simulink model "TP3_LABO_CONTROL_real_marcos"  (R2024b)
settings: Solver=VariableStepAuto  StartTime=0.0  StopTime=20  FixedStep=0.02  RelTol=1e-3
values from neighbouring files (symbols this model uses):
  Ad = eye(size(A)) + Ts * A    [observador_balta.m]    (also in observador_balta_2.m)
  Bd = Ts * B    [observador_balta.m]    (also in observador_balta_2.m)
  Cd = C    [observador_balta.m]    (also in observador_balta_2.m)
  K = K_scaled * T_inv    [real_estados_balta.m]    (also in todoslospuntos.m = -b * p / (1 - exp(-p * Ts)))
  L = P1*C    [estimacion_ecuaciones.m]    (also in observador_balta.m = P1*C1; observador_balta_2.m = P1*C1; real_estados_balta.m = T * L_scaled)
  Ts = 0.01    [Codigos_acomodados_14_5.m]    (also in PlantaEstable.m = median(diff(t_rec)); estimacion_ecuaciones.m; observador_balta.m = 0.02; observador_balta_2.m = 0.02)
undefined symbols (not defined in the file or in its folder): Kint
settings Model: Creator=lococ  LastModifiedBy=lococ

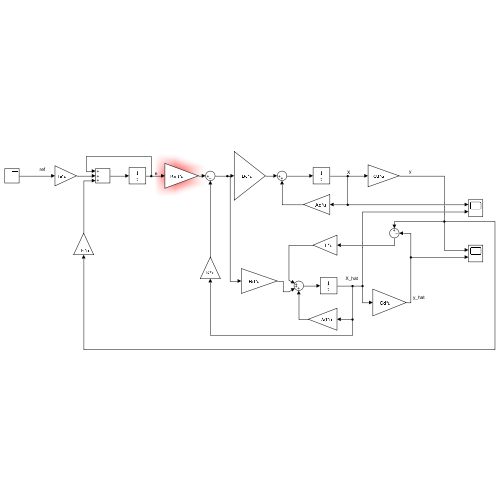
[thumbnail: Simulink's stored preview of the top-level diagram]
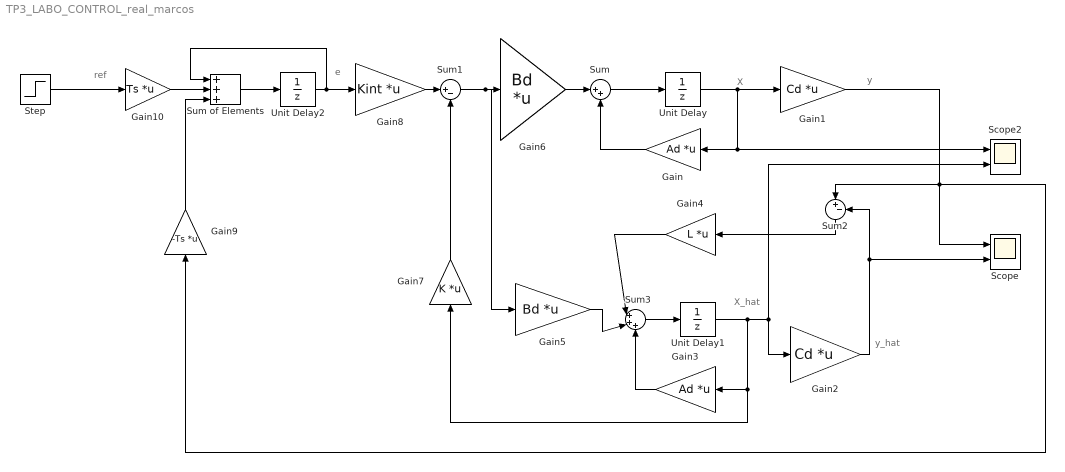
== system TP3_LABO_CONTROL_real_marcos ==
  note: ref
  note: e
  note: X_hat
  note: y_hat
  note: y
  note: X
  Gain : Gain  Gain=Ad  Multiplication=Matrix(K*u)
  Gain1 : Gain  Gain=Cd  Multiplication=Matrix(K*u)
  Gain10 : Gain  Gain=Ts  Multiplication=Matrix(K*u)
  Gain2 : Gain  Gain=Cd  Multiplication=Matrix(K*u)
  Gain3 : Gain  Gain=Ad  Multiplication=Matrix(K*u)
  Gain4 : Gain  Gain=L  Multiplication=Matrix(K*u)
  Gain5 : Gain  Gain=Bd  Multiplication=Matrix(K*u)
  Gain6 : Gain  Gain=Bd  Multiplication=Matrix(K*u)
  Gain7 : Gain  Gain=K  Multiplication=Matrix(K*u)
  Gain8 : Gain  Gain=Kint  Multiplication=Matrix(K*u)
  Gain9 : Gain  Gain=-Ts  Multiplication=Matrix(K*u)
  Scope : Scope  NumInputPorts=2
  Scope2 : Scope  NumInputPorts=2
  Step : Step  Time=[1;1]  Before=[0;0]  After=[30;0]  SampleTime=0  VectorParams1D=off
  Sum : Sum  Inputs=|++
  Sum of Elements : Sum  Inputs=+++
  Sum1 : Sum  Inputs=|+-
  Sum2 : Sum  Inputs=|+-
  Sum3 : Sum  Inputs=|+++
  Unit Delay : UnitDelay  SampleTime=0.02  HasFrameUpgradeWarning=on
  Unit Delay1 : UnitDelay  SampleTime=0.02  HasFrameUpgradeWarning=on
  Unit Delay2 : UnitDelay  SampleTime=0.02  HasFrameUpgradeWarning=on
  wires:
  Sum/1 -> Unit Delay/1
  Gain/1 -> Sum/2
  Unit Delay/1 -> Scope2/1, Gain/1, Gain1/1
  Gain2/1 -> Sum2/2, Scope/2
  Sum2/1 -> Gain4/1
  Gain4/1 -> Sum3/1
  Gain3/1 -> Sum3/3
  Gain5/1 -> Sum3/2
  Gain6/1 -> Sum/1
  Sum1/1 -> Gain5/1, Gain6/1
  Gain7/1 -> Sum1/2
  Gain1/1 -> Sum2/1, Gain9/1, Scope/1
  Sum3/1 -> Unit Delay1/1
  Unit Delay1/1 -> Gain2/1, Scope2/2, Gain7/1, Gain3/1
  Gain8/1 -> Sum1/1
  Unit Delay2/1 -> Sum of Elements/1, Gain8/1
  Sum of Elements/1 -> Unit Delay2/1
  Gain9/1 -> Sum of Elements/3
  Gain10/1 -> Sum of Elements/2
  Step/1 -> Gain10/1
